simulink model "parallel_modules_2_parasitic"  (R2023b)
settings: Solver=FixedStepDiscrete  StartTime=0.0  StopTime=Tfinal  FixedStep=SampleTime  RelTol=1e-3
InitFcn:
  | param
values from neighbouring files (symbols this model uses):
  ffund = 500    [param.m]
  Lload1 = 500e-6    (= 0.0005)    [param.m]
  Module1Phase = 0    [param.m]
  Rload1 = 0.1    [param.m]
  SampleTime = 1e-6    (= 1e-06)    [param.m]
  Vdc = 1200    [param.m]
libraries: simulink x14, spsMosfetLib x12, spsGroundLib x4, spsSeriesRLCBranchLib x3, spsVoltageMeasurementLib x3, spsCurrentMeasurementLib x3, BoomBox x3, spsDCVoltageSourceLib x2, dspstat3 x2, slpidlib x2, spsTriangleGeneratorLib x2, spsPower3phInstantaneousLib x1
settings Model: Creator=enes_  LastModifiedBy=enesa
settings SolverCC: AlgebraicLoopSolver=TrustRegion
settings DataIOCC: ReturnWorkspaceOutputs=off
settings DebuggingCC: UnconnectedInputMsg=warning  UnconnectedOutputMsg=warning  UnconnectedLineMsg=warning  ArithmeticOperatorsInVariantConditions=warning
settings ModelReferenceCC: EnableRefExpFcnMdlSchedulingChecks=on
settings SFSimCC: SimUseLocalCustomCode=off  CustomCodeUndefinedFunction=UseInterfaceOnly
settings RTWCC: RTWUseLocalCustomCode=off

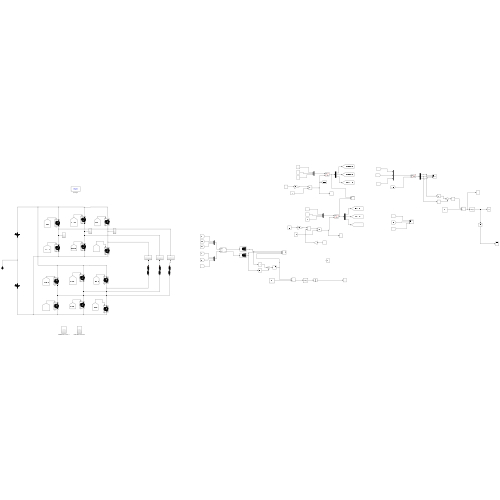
[thumbnail: Simulink's stored preview of the top-level diagram]
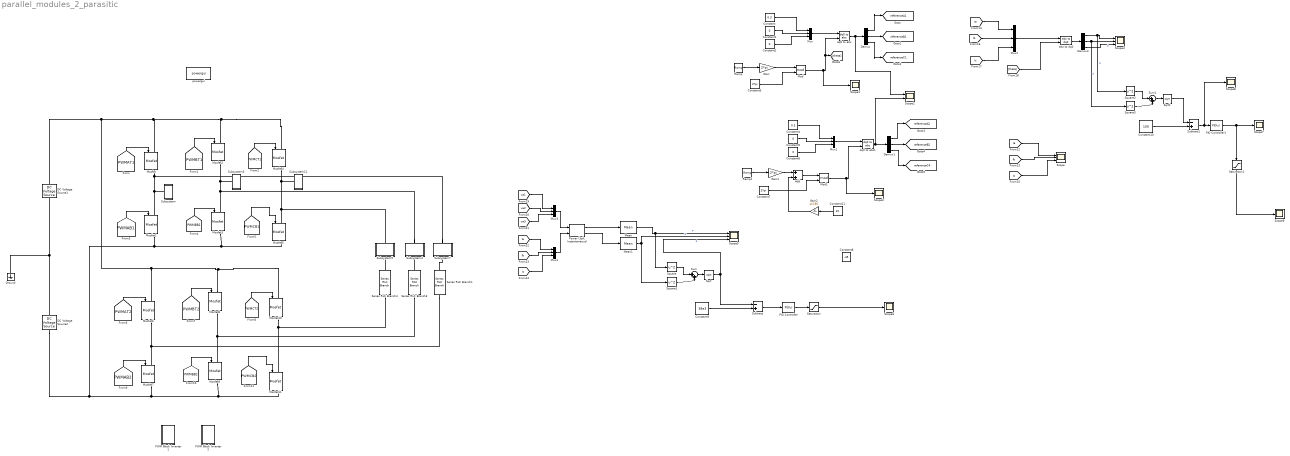
== system parallel_modules_2_parasitic ==
  Add : Sum
  Constant : Constant  Value=0.3
  Constant{1..2,5..6} (4 alike) : Constant  Value=0
  Constant10 : Constant  Value=100
  Constant11 : Constant  Value=10
  Constant3 : Constant  Value=2*pi
  Constant4 : Constant  Value=0.3
  Constant7 : Constant  Value=2*pi
  Constant8 : Constant  Value=-45
  Constant9 : Constant  Value=38e3
  DC Voltage Source1 : spsDCVoltageSourceLib/DC Voltage Source  Amplitude=Vdc/2  Measurements=None
  DC Voltage Source2 : spsDCVoltageSourceLib/DC Voltage Source  Amplitude=Vdc/2  Measurements=None
  Demux : Demux  Outputs=3
  Demux1 : Demux  Outputs=3
  Demux2 : Demux  Outputs=3
  Gain : Gain  Gain=2*pi
  Gain1 : Gain  Gain=2*pi
  Gain2 : Gain  Gain=pi/180
  Ground : spsGroundLib/Ground  LConnTagsString=a
  Mean : dspstat3/Mean  run=on  InputProcessing=Columns as channels (frame based)  reset_popup=None  directionMode=Each column  dimension=1  roiEnable=off  roiType=Rectangles  roiPortion=Entire ROI  roiOutput=Individual statistics for each ROI  roiFlag=off  roundingMode=Floor  overflowMode=off  outputDataTypeStr=Inherit: Same as accumulator  outputMin=[]  outputMax=[]  outputLastDataTypeStr=Inherit: Same as accumulator
  Mean1 : dspstat3/Mean  run=on  InputProcessing=Columns as channels (frame based)  reset_popup=None  directionMode=Each column  dimension=1  roiEnable=off  roiType=Rectangles  roiPortion=Entire ROI  roiOutput=Individual statistics for each ROI  roiFlag=off  roundingMode=Floor  overflowMode=off  outputDataTypeStr=Inherit: Same as accumulator  outputMin=[]  outputMax=[]  outputLastDataTypeStr=Inherit: Same as accumulator
  Mod : Math  Operator=mod
  Mod1 : Math  Operator=mod
  Mosfet{,1..11} (12 alike) : spsMosfetLib/Mosfet  Ron=0.1  Lon=0  Rd=0.01  Vfd=0  IC=0  Rs=1e5  Cs=inf  Measurements=on
  Mux{,1..4} (5 alike) : Mux  Inputs=3
  PID Controller : slpidlib/PID Controller  Controller=PID  Form=Parallel  TimeDomain=Discrete-time  UseExternalTs=off  SampleTime=1/ffund  IntegratorMethod=Forward Euler  FilterMethod=Forward Euler  ControllerParametersSource=internal  P=0.05  I=0  UseKiTs=off  D=0  N=100  UseFilter=on  TunerSelectOption=Transfer Function Based (PID Tuner App)  InitialConditionSource=internal  InitialConditionForIntegrator=0  InitialConditionForFilter=0  DifferentiatorICPrevScaledInput=0  ExternalReset=none  TrackingMode=off  Kt=1  LimitOutput=off  SatLimitsSource=internal  UpperSaturationLimit=inf  LowerSaturationLimit=-inf  LinearizeAsGain=on  AntiWindupMode=none  Kb=1  LimitIntegrator=off  UpperIntegratorSaturationLimit=inf  LowerIntegratorSaturationLimit=-inf  POutMin=[]  POutMax=[]  IOutMin=[]  IOutMax=[]  DOutMin=[]  DOutMax=[]  NOutMin=[]  NOutMax=[]  SumOutMin=[]  SumOutMax=[]  SaturationOutMin=[]  SaturationOutMax=[]  PParamMin=[]  PParamMax=[]  IParamMin=[]  IParamMax=[]  DParamMin=[]  DParamMax=[]  NParamMin=[]  NParamMax=[]  KbParamMin=[]  KbParamMax=[]  KtParamMin=[]  KtParamMax=[]  KbOutMin=[]  KbOutMax=[]  KtOutMin=[]  KtOutMax=[]  IntegratorOutMin=[]  IntegratorOutMax=[]  FilterOutMin=[]  FilterOutMax=[]  SumI1OutMin=[]  SumI1OutMax=[]  SumI2OutMin=[]  SumI2OutMax=[]  SumI3OutMin=[]  SumI3OutMax=[]  SumI4OutMin=[]  SumI4OutMax=[]  SumDOutMin=[]  SumDOutMax=[]  DifferentiatorOutMin=[]  DifferentiatorOutMax=[]  FilterDiffOutCoefMin=[]  FilterDiffOutCoefMax=[]  ReciprocalOutMin=[]  ReciprocalOutMax=[]  SumDenOutMin=[]  SumDenOutMax=[]  SumNumOutMin=[]  SumNumOutMax=[]  DivideOutMin=[]  DivideOutMax=[]  UdiffTsProdOutMin=[]  UdiffTsProdOutMax=[]  NTsProdOutMin=[]  NTsProdOutMax=[]  UintegralTsProdOutMin=[]  UintegralTsProdOutMax=[]  UngainTsProdOutMin=[]  UngainTsProdOutMax=[]  ClampingZeroOutDataTypeStr=Inherit: Inherit via back propagation  ClampingZeroOutMin=[]  ClampingZeroOutMax=[]  FilterDenConstantOutDataTypeStr=Inherit: Inherit via back propagation  FilterDenConstantOutMin=[]  FilterDenConstantOutMax=[]  PCopyOutDataTypeStr=Inherit: Inherit via back propagation  PCopyOutMin=[]  PCopyOutMax=[]  NCopyOutDataTypeStr=Inherit: Inherit via back propagation  NCopyOutMin=[]  NCopyOutMax=[]  IntegratorContinuousStateAttributes=''  IntegratorStateMustResolveToSignalObject=off  IntegratorRTWStateStorageClass=Auto  FilterContinuousStateAttributes=''  FilterStateMustResolveToSignalObject=off  FilterRTWStateStorageClass=Auto  ParallelPVariant=InternalParameters  IdealPVariant=Disabled  IVariant=InternalParameters  DVariant=InternalParameters  IntegratorVariant=Discrete  SatVariant=Disabled  AWVariant=Passthrough  PCopyVariant=Disabled  TRVariant=Disabled  FdbkBlocksVariant=Forward  IdealPFdbkVariant=Disabled  SatFdbkVariant=Disabled  DerivativeFilterVariant=ForwardEulerFilter  NVariant=InternalParameters  NCopyVariant=Disabled  FilterICVariant=InternalICsFilter  IntegratorICVariant=InternalICs  ExternalResetVariant=Disabled  TRSumVariant=Passthrough  SumFdbkVariant=Disabled  SumVariant=Sum_PID  TsampFilterVariant=InternalTs  TsampNgainVariant=Passthrough  TsampIntegralVariant=Disabled_SignalSpec  ExternalSaturationOutDataTypeStr=Inherit: Same as second input
  PID Controller1 : slpidlib/PID Controller  Controller=PID  Form=Parallel  TimeDomain=Discrete-time  UseExternalTs=off  SampleTime=1/ffund  IntegratorMethod=Forward Euler  FilterMethod=Forward Euler  ControllerParametersSource=internal  P=0.5  I=0.05  UseKiTs=off  D=0  N=100  UseFilter=on  TunerSelectOption=Transfer Function Based (PID Tuner App)  InitialConditionSource=internal  InitialConditionForIntegrator=0  InitialConditionForFilter=0  DifferentiatorICPrevScaledInput=0  ExternalReset=none  TrackingMode=off  Kt=1  LimitOutput=off  SatLimitsSource=internal  UpperSaturationLimit=inf  LowerSaturationLimit=-inf  LinearizeAsGain=on  AntiWindupMode=none  Kb=1  LimitIntegrator=off  UpperIntegratorSaturationLimit=inf  LowerIntegratorSaturationLimit=-inf  POutMin=[]  POutMax=[]  IOutMin=[]  IOutMax=[]  DOutMin=[]  DOutMax=[]  NOutMin=[]  NOutMax=[]  SumOutMin=[]  SumOutMax=[]  SaturationOutMin=[]  SaturationOutMax=[]  PParamMin=[]  PParamMax=[]  IParamMin=[]  IParamMax=[]  DParamMin=[]  DParamMax=[]  NParamMin=[]  NParamMax=[]  KbParamMin=[]  KbParamMax=[]  KtParamMin=[]  KtParamMax=[]  KbOutMin=[]  KbOutMax=[]  KtOutMin=[]  KtOutMax=[]  IntegratorOutMin=[]  IntegratorOutMax=[]  FilterOutMin=[]  FilterOutMax=[]  SumI1OutMin=[]  SumI1OutMax=[]  SumI2OutMin=[]  SumI2OutMax=[]  SumI3OutMin=[]  SumI3OutMax=[]  SumI4OutMin=[]  SumI4OutMax=[]  SumDOutMin=[]  SumDOutMax=[]  DifferentiatorOutMin=[]  DifferentiatorOutMax=[]  FilterDiffOutCoefMin=[]  FilterDiffOutCoefMax=[]  ReciprocalOutMin=[]  ReciprocalOutMax=[]  SumDenOutMin=[]  SumDenOutMax=[]  SumNumOutMin=[]  SumNumOutMax=[]  DivideOutMin=[]  DivideOutMax=[]  UdiffTsProdOutMin=[]  UdiffTsProdOutMax=[]  NTsProdOutMin=[]  NTsProdOutMax=[]  UintegralTsProdOutMin=[]  UintegralTsProdOutMax=[]  UngainTsProdOutMin=[]  UngainTsProdOutMax=[]  ClampingZeroOutDataTypeStr=Inherit: Inherit via back propagation  ClampingZeroOutMin=[]  ClampingZeroOutMax=[]  FilterDenConstantOutDataTypeStr=Inherit: Inherit via back propagation  FilterDenConstantOutMin=[]  FilterDenConstantOutMax=[]  PCopyOutDataTypeStr=Inherit: Inherit via back propagation  PCopyOutMin=[]  PCopyOutMax=[]  NCopyOutDataTypeStr=Inherit: Inherit via back propagation  NCopyOutMin=[]  NCopyOutMax=[]  IntegratorContinuousStateAttributes=''  IntegratorStateMustResolveToSignalObject=off  IntegratorRTWStateStorageClass=Auto  FilterContinuousStateAttributes=''  FilterStateMustResolveToSignalObject=off  FilterRTWStateStorageClass=Auto  ParallelPVariant=InternalParameters  IdealPVariant=Disabled  IVariant=InternalParameters  DVariant=InternalParameters  IntegratorVariant=Discrete  SatVariant=Disabled  AWVariant=Passthrough  PCopyVariant=Disabled  TRVariant=Disabled  FdbkBlocksVariant=Forward  IdealPFdbkVariant=Disabled  SatFdbkVariant=Disabled  DerivativeFilterVariant=ForwardEulerFilter  NVariant=InternalParameters  NCopyVariant=Disabled  FilterICVariant=InternalICsFilter  IntegratorICVariant=InternalICs  ExternalResetVariant=Disabled  TRSumVariant=Passthrough  SumFdbkVariant=Disabled  SumVariant=Sum_PID  TsampFilterVariant=InternalTs  TsampNgainVariant=Passthrough  TsampIntegralVariant=Disabled_SignalSpec  ExternalSaturationOutDataTypeStr=Inherit: Same as second input
  PWM Block Inverter 1 : Subsystem
  PWM Block Inverter 2 : Subsystem
  "Power (3ph, Instantaneous)" : spsPower3phInstantaneousLib/Power (3ph, Instantaneous)
  Ramp : simulink/Sources/Ramp  slope=ffund  start=0  InitialOutput=0
  Ramp1 : simulink/Sources/Ramp  slope=ffund  start=0  InitialOutput=0
  Saturation : Saturate  UpperLimit=90  LowerLimit=0
  Saturation1 : Saturate  UpperLimit=90  LowerLimit=0
  Scope : Scope  NumInputPorts=3
  Scope{1,3,6..9} (6 alike) : Scope
  Scope2 : Scope  NumInputPorts=2
  Scope4 : Scope  NumInputPorts=3
  Scope5 : Scope  NumInputPorts=3
  Series RLC Branch1 : spsSeriesRLCBranchLib/Series RLC Branch  LConnTagsString=__new0  RConnTagsString=__new0  BranchType=RL  Resistance=Rload1  Inductance=Lload1  SetiL0=off  InitialCurrent=0  Capacitance=1e-6  Setx0=off  InitialVoltage=0  Measurements=None
  Series RLC Branch3 : spsSeriesRLCBranchLib/Series RLC Branch  LConnTagsString=__new0  RConnTagsString=__new0  BranchType=RL  Resistance=Rload1  Inductance=Lload1  SetiL0=off  InitialCurrent=0  Capacitance=1e-6  Setx0=off  InitialVoltage=0  Measurements=None
  Series RLC Branch4 : spsSeriesRLCBranchLib/Series RLC Branch  LConnTagsString=__new0  RConnTagsString=__new0  BranchType=RL  Resistance=Rload1  Inductance=Lload1  SetiL0=off  InitialCurrent=0  Capacitance=1e-6  Setx0=off  InitialVoltage=0  Measurements=None
  Sqrt : Sqrt
  Sqrt1 : Sqrt
  Square{,1..3} (4 alike) : Math  Operator=square
  Subsystem : Subsystem
  Subsystem11 : Subsystem
  Subsystem3 : Subsystem
  Subsystem4 : Subsystem
  Subsystem5 : Subsystem
  Subsystem7 : Subsystem
  Subtract : Sum  Inputs=-+
  Subtract1 : Sum  Inputs=-+
  Sum : Sum  Inputs=|++
  Sum1 : Sum  Inputs=|++
  abc to dq0 : BoomBox/Transformations/abc to dq0  KBID=kb0601
      settings: SourceProductName=imperix blockset
  dq0 to abc : BoomBox/Transformations/dq0 to abc  KBID=kb0602
      settings: SourceProductName=imperix blockset
  dq0 to abc1 : BoomBox/Transformations/dq0 to abc  KBID=kb0602
      settings: SourceProductName=imperix blockset
  powergui : sps_lib/powergui  Priority=1  SimulationMode=Discrete  SampleTime=SampleTime  frequency=60  Iterations=50  frequencyindice=0  Pbase=100e6  ErrMax=1e-4  UnitsV=kV  UnitsW=MW  buscounter=0  FunctionMessages=off  echomessages=off  EnableUseOfTLC=off  CurrentSourceSwitches=off  DisableSnubberDevices=off  DisableRonSwitches=off  DisableVfSwitches=off  DisplayEquations=off  AutomaticDiscreteSolvers=off  SolverType=Tustin/Backward Euler (TBE)  Interpol=off  ExternalGateDelay=off  methode=off  Ts=100  x0status=blocks  SPID=off  SwTol=0  HookPort=off  NonlinearTolerance=1e-4  nMaxIteration=100  ContinueOnMaxIteration=off  RestoreLinks=warning  ResistiveCurrentMeasurement=off  Frange=[0:2:500]  Ylog=off  Xlog=on  ShowGrid=off  save=off  variable=ZData  structure=0  ZoomFFT=off  StartTime=0.0  cycles=1  DisplayStyle=1  fundamental=60  FreqAxis=off  MaxFrequency=1000  frequencyindicesteady=1  RmsSteady=1  display=off
  tag scope: referenceA1=global, referenceA2=global, referenceB1=global, referenceB2=global, referenceC1=global, referenceC4=global
  wires:
  [PWMBB1] -> Mosfet3/1
  [PWMCB1] -> Mosfet5/1
  [PWMAB1] -> Mosfet1/1
  [PWMBT1] -> Mosfet2/1
  [PWMCT1] -> Mosfet4/1
  [PWMAT1] -> Mosfet/1
  [PWMAT2] -> Mosfet6/1
  [PWMCT2] -> Mosfet10/1
  [PWMBT2] -> Mosfet8/1
  [PWMCB2] -> Mosfet11/1
  [PWMAB2] -> Mosfet7/1
  [PWMBB2] -> Mosfet9/1
  Constant/1 -> Mux/1
  Constant1/1 -> Mux/2
  Constant2/1 -> Mux/3
  Mux/1 -> dq0 to abc/1
  Constant3/1 -> Mod/2
  Mod/1 -> Scope1/1, [theta], dq0 to abc/2
  dq0 to abc/1 -> Scope2/1, Demux/1
  Gain/1 -> Mod/1
  Ramp/1 -> Gain/1
  Constant6/1 -> Mux1/3
  Constant7/1 -> Mod1/2
  Mux1/1 -> dq0 to abc1/1
  Mod1/1 -> Scope3/1, dq0 to abc1/2
  Constant4/1 -> Mux1/1
  Constant5/1 -> Mux1/2
  Ramp1/1 -> Gain1/1
  Gain1/1 -> Add/1
  Add/1 -> Mod1/1
  Gain2/1 -> Add/2
  Demux/1 -> [referenceA1]
  Demux/2 -> [referenceB1]
  Demux/3 -> [referenceC1]
  Demux1/1 -> [referenceA2]
  Demux1/2 -> [referenceB2]
  Demux1/3 -> [referenceC4]
  dq0 to abc1/1 -> Scope2/2, Demux1/1
  [Ia] -> Scope/1
  [Ib] -> Scope/2
  [Ic] -> Scope/3
  Mux2/1 -> abc to dq0/1
  abc to dq0/1 -> Demux2/1
  [theta] -> abc to dq0/2
  [Ia] -> Mux2/1
  [Ib] -> Mux2/2
  [Ic] -> Mux2/3
  Demux2/1 -> Square2/1, Scope4/1  "d"
  Demux2/2 -> Square3/1, Scope4/2  "q"
  Demux2/3 -> Scope4/3  "0"
  [va1] -> Mux3/1
  [va2] -> Mux3/2
  [va3] -> Mux3/3
  Mux3/1 -> "Power (3ph, Instantaneous)"/1
  Mux4/1 -> "Power (3ph, Instantaneous)"/2
  [Ia] -> Mux4/1
  [Ib] -> Mux4/2
  [Ic] -> Mux4/3
  "Power (3ph, Instantaneous)"/1 -> Mean/1
  "Power (3ph, Instantaneous)"/2 -> Mean1/1
  Mean/1 -> Square/1, Scope5/1  "P"
  Mean1/1 -> Square1/1, Scope5/2  "Q"
  Square/1 -> Sum/1
  Square1/1 -> Sum/2
  Sum/1 -> Sqrt/1
  Sqrt/1 -> Scope5/3, Subtract/1  "S"
  Constant9/1 -> Subtract/2
  Subtract/1 -> PID Controller/1
  PID Controller/1 -> Saturation/1
  Saturation/1 -> Scope6/1
  Square2/1 -> Sum1/1
  Sum1/1 -> Sqrt1/1
  Square3/1 -> Sum1/2
  Constant10/1 -> Subtract1/2
  Subtract1/1 -> Scope8/1, PID Controller1/1
  Sqrt1/1 -> Subtract1/1
  PID Controller1/1 -> Scope7/1, Saturation1/1
  Saturation1/1 -> Scope9/1
  Constant11/1 -> Gain2/1
  connections:
  Series RLC Branch3/LConn1 -- Subsystem4/LConn1
  Series RLC Branch4/LConn1 -- Subsystem5/LConn1
  Mosfet2/RConn1 -- Subsystem3/LConn1 -- Subsystem4/RConn1 -- Mosfet3/LConn1
  Mosfet4/RConn1 -- Subsystem11/LConn1 -- Subsystem5/RConn1 -- Mosfet5/LConn1
  Mosfet11/RConn1 -- Mosfet9/RConn1 -- DC Voltage Source2/LConn1 -- Mosfet1/RConn1 -- Mosfet3/RConn1 -- Mosfet5/RConn1 -- Mosfet7/RConn1
  Mosfet/RConn1 -- Subsystem/LConn1 -- Mosfet1/LConn1 -- Subsystem7/RConn1
  Mosfet6/LConn1 -- Mosfet/LConn1 -- Mosfet2/LConn1 -- Mosfet4/LConn1 -- DC Voltage Source1/RConn1 -- Mosfet10/LConn1 -- Mosfet8/LConn1
  Mosfet6/RConn1 -- Mosfet7/LConn1 -- Series RLC Branch1/RConn1
  Mosfet8/RConn1 -- Series RLC Branch3/RConn1 -- Mosfet9/LConn1
  Mosfet10/RConn1 -- Series RLC Branch4/RConn1 -- Mosfet11/LConn1
  Series RLC Branch1/LConn1 -- Subsystem7/LConn1
  DC Voltage Source2/RConn1 -- Ground/LConn1 -- DC Voltage Source1/LConn1

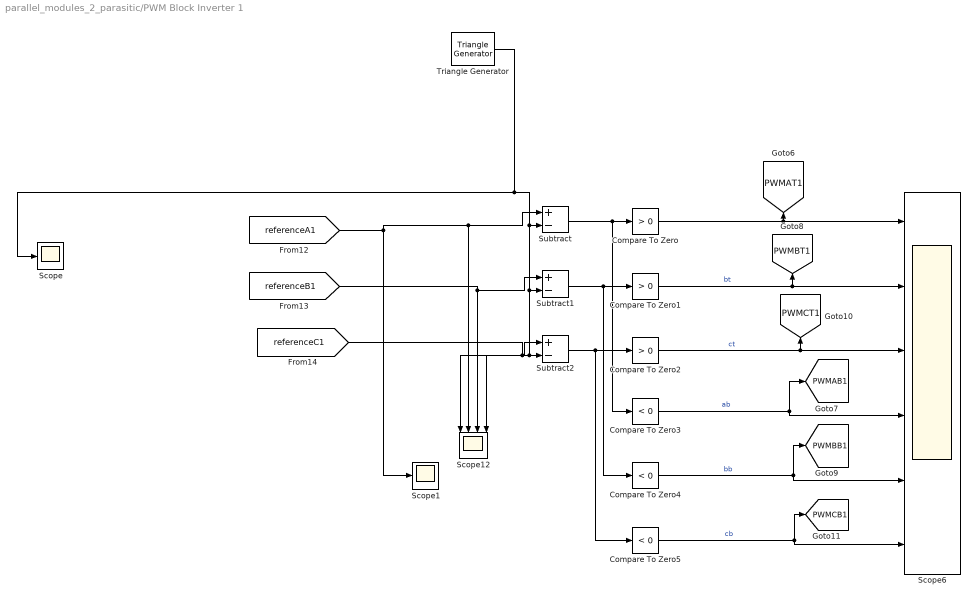
== system parallel_modules_2_parasitic/PWM Block Inverter 1 ==
  Compare To Zero : simulink/Logic and Bit Operations/Compare To Zero  relop=>  OutDataTypeStr=boolean
  Compare To Zero1 : simulink/Logic and Bit Operations/Compare To Zero  relop=>  OutDataTypeStr=boolean
  Compare To Zero2 : simulink/Logic and Bit Operations/Compare To Zero  relop=>  OutDataTypeStr=boolean
  Compare To Zero3 : simulink/Logic and Bit Operations/Compare To Zero  relop=<  OutDataTypeStr=boolean
  Compare To Zero4 : simulink/Logic and Bit Operations/Compare To Zero  relop=<  OutDataTypeStr=boolean
  Compare To Zero5 : simulink/Logic and Bit Operations/Compare To Zero  relop=<  OutDataTypeStr=boolean
  Scope : Scope
  Scope1 : Scope
  Scope12 : Scope  NumInputPorts=4
  Scope6 : Scope  NumInputPorts=6
  Subtract : Sum  Inputs=+-
  Subtract1 : Sum  Inputs=+-
  Subtract2 : Sum  Inputs=+-
  Triangle Generator : spsTriangleGeneratorLib/Triangle Generator  Freq=fsw  Phase=Module1Phase  Ts=SampleTime
  tag scope: PWMAB1=global, PWMAT1=global, PWMBB1=global, PWMBT1=global, PWMCB1=global, PWMCT1=global
  wires:
  Compare To Zero2/1 -> [PWMCT1], Scope6/3  "ct"
  [referenceB1] -> Subtract1/1, Scope12/3
  Subtract2/1 -> Compare To Zero5/1, Compare To Zero2/1
  [referenceA1] -> Subtract/1, Scope12/2, Scope1/1
  Subtract1/1 -> Compare To Zero4/1, Compare To Zero1/1
  Triangle Generator/1 -> Scope12/1, Subtract2/2, Subtract1/2, Subtract/2, Scope/1
  Compare To Zero/1 -> Scope6/1, [PWMAT1]
  Subtract/1 -> Compare To Zero3/1, Compare To Zero/1
  Compare To Zero1/1 -> [PWMBT1], Scope6/2  "bt"
  Compare To Zero5/1 -> [PWMCB1], Scope6/6  "cb"
  Compare To Zero4/1 -> [PWMBB1], Scope6/5  "bb"
  [referenceC1] -> Scope12/4, Subtract2/1
  Compare To Zero3/1 -> [PWMAB1], Scope6/4  "ab"

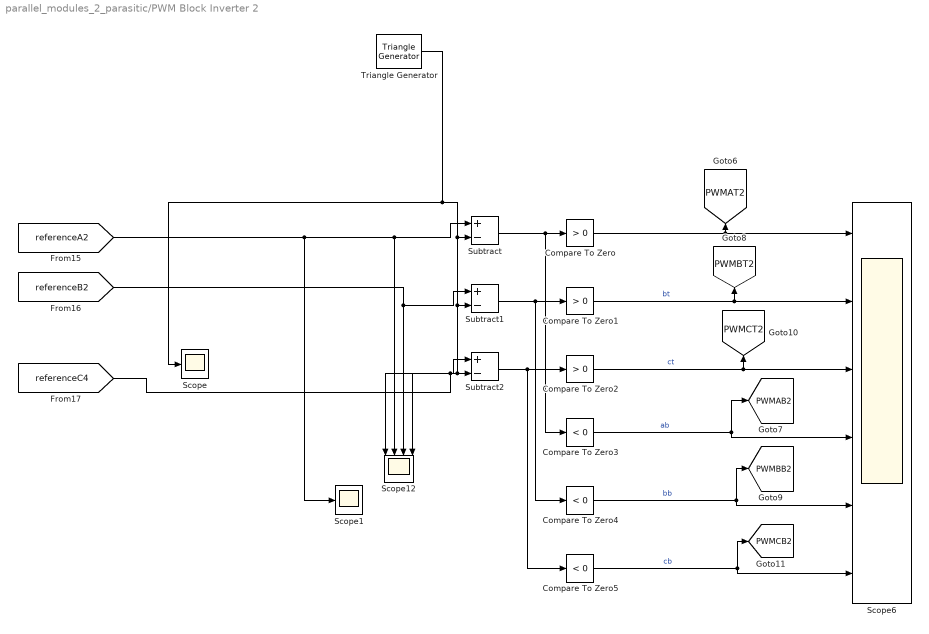
== system parallel_modules_2_parasitic/PWM Block Inverter 2 ==
  Compare To Zero : simulink/Logic and Bit Operations/Compare To Zero  relop=>  OutDataTypeStr=boolean
  Compare To Zero1 : simulink/Logic and Bit Operations/Compare To Zero  relop=>  OutDataTypeStr=boolean
  Compare To Zero2 : simulink/Logic and Bit Operations/Compare To Zero  relop=>  OutDataTypeStr=boolean
  Compare To Zero3 : simulink/Logic and Bit Operations/Compare To Zero  relop=<  OutDataTypeStr=boolean
  Compare To Zero4 : simulink/Logic and Bit Operations/Compare To Zero  relop=<  OutDataTypeStr=boolean
  Compare To Zero5 : simulink/Logic and Bit Operations/Compare To Zero  relop=<  OutDataTypeStr=boolean
  Scope : Scope
  Scope1 : Scope
  Scope12 : Scope  NumInputPorts=4
  Scope6 : Scope  NumInputPorts=6
  Subtract : Sum  Inputs=+-
  Subtract1 : Sum  Inputs=+-
  Subtract2 : Sum  Inputs=+-
  Triangle Generator : spsTriangleGeneratorLib/Triangle Generator  Freq=fsw  Phase=Module1Phase  Ts=SampleTime
  tag scope: PWMAB2=global, PWMAT2=global, PWMBB2=global, PWMBT2=global, PWMCB2=global, PWMCT2=global
  wires:
  Compare To Zero2/1 -> [PWMCT2], Scope6/3  "ct"
  [referenceB2] -> Subtract1/1, Scope12/3
  Subtract2/1 -> Compare To Zero5/1, Compare To Zero2/1
  [referenceA2] -> Scope1/1, Subtract/1, Scope12/2
  Subtract1/1 -> Compare To Zero4/1, Compare To Zero1/1
  Triangle Generator/1 -> Scope12/1, Subtract2/2, Subtract1/2, Subtract/2, Scope/1
  Compare To Zero/1 -> Scope6/1, [PWMAT2]
  Subtract/1 -> Compare To Zero3/1, Compare To Zero/1
  Compare To Zero1/1 -> [PWMBT2], Scope6/2  "bt"
  Compare To Zero5/1 -> [PWMCB2], Scope6/6  "cb"
  Compare To Zero4/1 -> [PWMBB2], Scope6/5  "bb"
  [referenceC4] -> Scope12/4, Subtract2/1
  Compare To Zero3/1 -> [PWMAB2], Scope6/4  "ab"

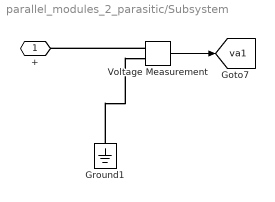
== system parallel_modules_2_parasitic/Subsystem ==
  Ground1 : spsGroundLib/Ground  LConnTagsString=a
  Voltage Measurement : spsVoltageMeasurementLib/Voltage Measurement  PhasorSimulation=off  OutputType=Complex  PSBequivalent=0
  + : PMIOPort  Side=Left
  tag scope: va1=global
  wires:
  Voltage Measurement/1 -> [va1]
  connections:
  Voltage Measurement/LConn1 -- +/RConn1
  Ground1/LConn1 -- Voltage Measurement/LConn2

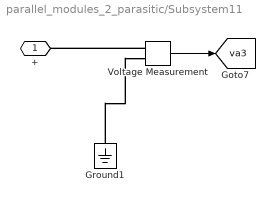
== system parallel_modules_2_parasitic/Subsystem11 ==
  Ground1 : spsGroundLib/Ground  LConnTagsString=a
  Voltage Measurement : spsVoltageMeasurementLib/Voltage Measurement  PhasorSimulation=off  OutputType=Complex  PSBequivalent=0
  + : PMIOPort  Side=Left
  tag scope: va3=global
  wires:
  Voltage Measurement/1 -> [va3]
  connections:
  Voltage Measurement/LConn1 -- +/RConn1
  Ground1/LConn1 -- Voltage Measurement/LConn2

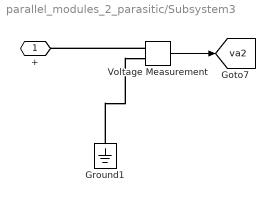
== system parallel_modules_2_parasitic/Subsystem3 ==
  Ground1 : spsGroundLib/Ground  LConnTagsString=a
  Voltage Measurement : spsVoltageMeasurementLib/Voltage Measurement  PhasorSimulation=off  OutputType=Complex  PSBequivalent=0
  + : PMIOPort  Side=Left
  tag scope: va2=global
  wires:
  Voltage Measurement/1 -> [va2]
  connections:
  Voltage Measurement/LConn1 -- +/RConn1
  Ground1/LConn1 -- Voltage Measurement/LConn2

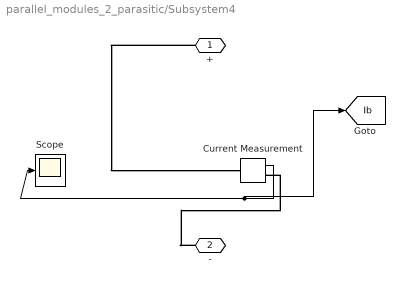
== system parallel_modules_2_parasitic/Subsystem4 ==
  Current Measurement : spsCurrentMeasurementLib/Current Measurement  PhasorSimulation=off  OutputType=Complex  PSBequivalent=0
  Scope : Scope
  + : PMIOPort  Side=Right
  - : PMIOPort  Port=2  Side=Left
  tag scope: Ib=global
  wires:
  Current Measurement/1 -> [Ib], Scope/1
  connections:
  +/RConn1 -- Current Measurement/LConn1
  -/RConn1 -- Current Measurement/RConn1

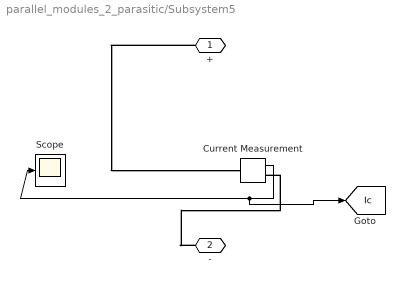
== system parallel_modules_2_parasitic/Subsystem5 ==
  Current Measurement : spsCurrentMeasurementLib/Current Measurement  PhasorSimulation=off  OutputType=Complex  PSBequivalent=0
  Scope : Scope
  + : PMIOPort  Side=Right
  - : PMIOPort  Port=2  Side=Left
  tag scope: Ic=global
  wires:
  Current Measurement/1 -> Scope/1, [Ic]
  connections:
  +/RConn1 -- Current Measurement/LConn1
  -/RConn1 -- Current Measurement/RConn1

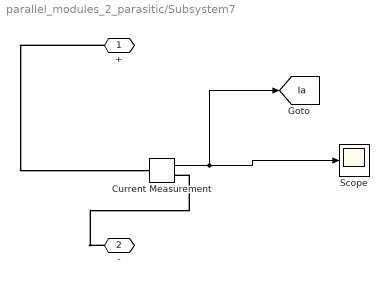
== system parallel_modules_2_parasitic/Subsystem7 ==
  Current Measurement : spsCurrentMeasurementLib/Current Measurement  PhasorSimulation=off  OutputType=Complex  PSBequivalent=0
  Scope : Scope
  + : PMIOPort  Side=Right
  - : PMIOPort  Port=2  Side=Left
  tag scope: Ia=global
  wires:
  Current Measurement/1 -> [Ia], Scope/1
  connections:
  +/RConn1 -- Current Measurement/LConn1
  -/RConn1 -- Current Measurement/RConn1
